simulink model "final_heart_sym2_level4_fixed"  (R2021a)
settings: Solver=VariableStepAuto  StartTime=0.0  StopTime=8  RelTol=1e-3
undefined symbols (not defined in the file or in its folder): lambda2
libraries: dspsigops x1, dspquant2 x1
(part 1 of 2)
settings Model: Creator=Ruth Matienzo  LastModifiedBy=Acer

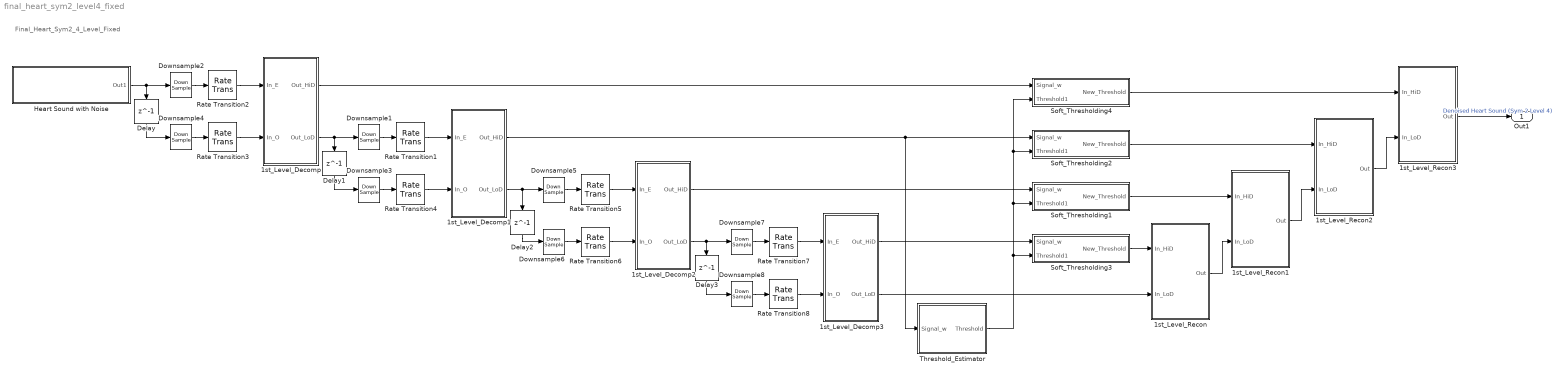
== system final_heart_sym2_level4_fixed ==
  note: Final_Heart_Sym2_4_Level_Fixed
  1st_Level_Decomp : Subsystem
  1st_Level_Decomp1 : Subsystem
  1st_Level_Decomp2 : Subsystem
  1st_Level_Decomp3 : Subsystem
  1st_Level_Recon : Subsystem
  1st_Level_Recon1 : Subsystem
  1st_Level_Recon2 : Subsystem
  1st_Level_Recon3 : Subsystem
  Delay{,1..3} (4 alike) : Delay  DelayLength=1  SampleTime=1/44100
  Downsample{1..8} (8 alike) : DownSample  N=30  RateOptions=Allow multirate processing
  Heart Sound with Noise : Subsystem
  Rate Transition{1..8} (8 alike) : RateTransition
  Soft_Thresholding1 : Subsystem
  Soft_Thresholding2 : Subsystem
  Soft_Thresholding3 : Subsystem
  Soft_Thresholding4 : Subsystem
  Threshold_Estimator : Subsystem
  Out1 : Outport  OutDataTypeStr=double  SampleTime=1/44100
  wires:
  1st_Level_Decomp1/1(Out_HiD) -> Soft_Thresholding2/1(Signal_w), Threshold_Estimator/1(Signal_w)
  1st_Level_Decomp/1(Out_HiD) -> Soft_Thresholding4/1(Signal_w)
  Delay1/1 -> Downsample3/1
  1st_Level_Decomp/2(Out_LoD) -> Downsample1/1, Delay1/1
  1st_Level_Decomp1/2(Out_LoD) -> Downsample5/1, Delay2/1
  Delay2/1 -> Downsample6/1
  Soft_Thresholding1/1(New_Threshold) -> 1st_Level_Recon1/1(In_HiD)
  1st_Level_Recon1/1(Out) -> 1st_Level_Recon2/2(In_LoD)
  1st_Level_Recon2/1(Out) -> 1st_Level_Recon3/2(In_LoD)
  Soft_Thresholding4/1(New_Threshold) -> 1st_Level_Recon3/1(In_HiD)
  Soft_Thresholding2/1(New_Threshold) -> 1st_Level_Recon2/1(In_HiD)
  Delay3/1 -> Downsample8/1
  1st_Level_Decomp2/1(Out_HiD) -> Soft_Thresholding1/1(Signal_w)
  1st_Level_Decomp3/1(Out_HiD) -> Soft_Thresholding3/1(Signal_w)
  Soft_Thresholding3/1(New_Threshold) -> 1st_Level_Recon/1(In_HiD)
  1st_Level_Decomp3/2(Out_LoD) -> 1st_Level_Recon/2(In_LoD)
  1st_Level_Recon/1(Out) -> 1st_Level_Recon1/2(In_LoD)
  Threshold_Estimator/1(Threshold) -> Soft_Thresholding3/2(Threshold1), Soft_Thresholding1/2(Threshold1), Soft_Thresholding4/2(Threshold1), Soft_Thresholding2/2(Threshold1)
  1st_Level_Decomp2/2(Out_LoD) -> Downsample7/1, Delay3/1
  1st_Level_Recon3/1(Out) -> Out1/1  "Denoised Heart Sound (Sym 2 Level 4)"
  Rate Transition2/1 -> 1st_Level_Decomp/1(In_E)
  Downsample2/1 -> Rate Transition2/1
  Rate Transition3/1 -> 1st_Level_Decomp/2(In_O)
  Delay/1 -> Downsample4/1
  Downsample4/1 -> Rate Transition3/1
  Heart Sound with Noise/1(Out1) -> Delay/1, Downsample2/1
  Rate Transition1/1 -> 1st_Level_Decomp1/1(In_E)
  Downsample1/1 -> Rate Transition1/1
  Rate Transition4/1 -> 1st_Level_Decomp1/2(In_O)
  Downsample3/1 -> Rate Transition4/1
  Rate Transition5/1 -> 1st_Level_Decomp2/1(In_E)
  Rate Transition6/1 -> 1st_Level_Decomp2/2(In_O)
  Downsample5/1 -> Rate Transition5/1
  Downsample6/1 -> Rate Transition6/1
  Rate Transition7/1 -> 1st_Level_Decomp3/1(In_E)
  Rate Transition8/1 -> 1st_Level_Decomp3/2(In_O)
  Downsample7/1 -> Rate Transition7/1
  Downsample8/1 -> Rate Transition8/1

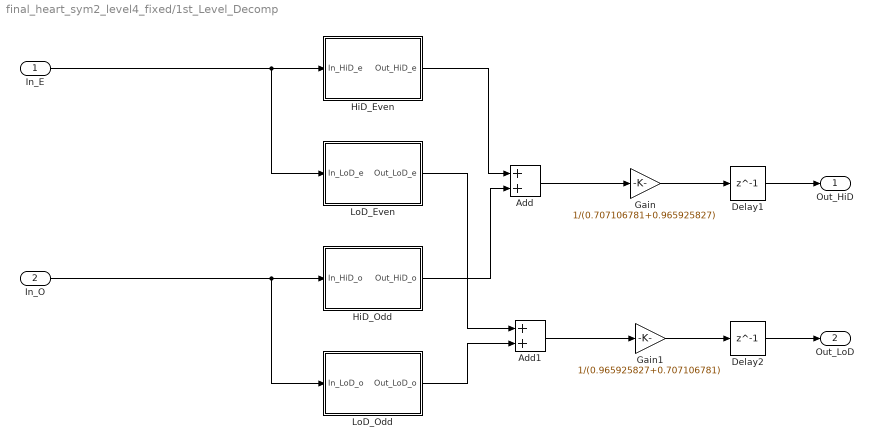
== system final_heart_sym2_level4_fixed/1st_Level_Decomp ==
  In_E : Inport  OutDataTypeStr=double  SampleTime=1/44100
  In_O : Inport  Port=2  OutDataTypeStr=double  SampleTime=1/44100
  Add : Sum  AccumDataTypeStr=double  OutDataTypeStr=double
  Add1 : Sum  AccumDataTypeStr=double  OutDataTypeStr=double
  Delay1 : Delay  DelayLength=1  SampleTime=1/44100
  Delay2 : Delay  DelayLength=1  SampleTime=1/44100
  Gain : Gain  Gain=1/(0.707106781+0.965925827)  ParamDataTypeStr=double  OutDataTypeStr=double
  Gain1 : Gain  Gain=1/(0.965925827+0.707106781)  ParamDataTypeStr=double  OutDataTypeStr=double
  HiD_Even : Subsystem
  HiD_Odd : Subsystem
  LoD_Even : Subsystem
  LoD_Odd : Subsystem
  Out_HiD : Outport  OutDataTypeStr=double  SampleTime=1/44100
  Out_LoD : Outport  Port=2  OutDataTypeStr=double  SampleTime=1/44100
  wires:
  HiD_Even/1(Out_HiD_e) -> Add/1
  HiD_Odd/1(Out_HiD_o) -> Add/2
  LoD_Even/1(Out_LoD_e) -> Add1/1
  Delay1/1 -> Out_HiD/1
  Delay2/1 -> Out_LoD/1
  In_E/1 -> HiD_Even/1(In_HiD_e), LoD_Even/1(In_LoD_e)
  In_O/1 -> HiD_Odd/1(In_HiD_o), LoD_Odd/1(In_LoD_o)
  LoD_Odd/1(Out_LoD_o) -> Add1/2
  Gain/1 -> Delay1/1
  Add/1 -> Gain/1
  Gain1/1 -> Delay2/1
  Add1/1 -> Gain1/1

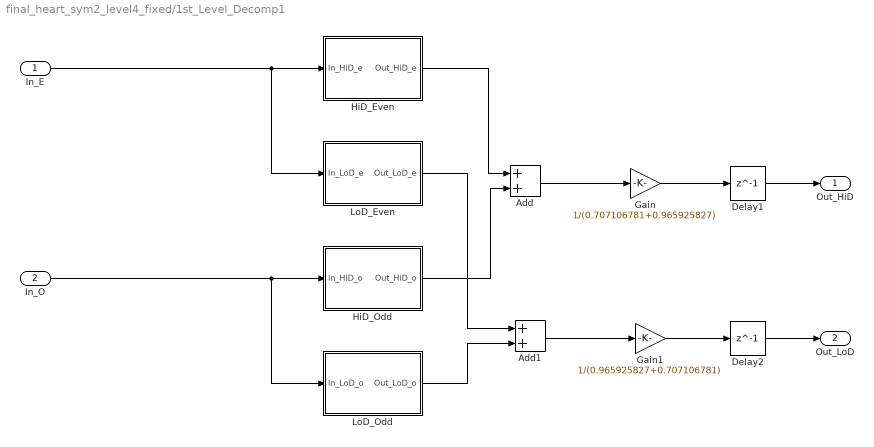
== system final_heart_sym2_level4_fixed/1st_Level_Decomp1 ==
  In_E : Inport  OutDataTypeStr=double  SampleTime=1/44100
  In_O : Inport  Port=2  OutDataTypeStr=double  SampleTime=1/44100
  Add : Sum  AccumDataTypeStr=double  OutDataTypeStr=double
  Add1 : Sum  AccumDataTypeStr=double  OutDataTypeStr=double
  Delay1 : Delay  DelayLength=1  SampleTime=1/44100
  Delay2 : Delay  DelayLength=1  SampleTime=1/44100
  Gain : Gain  Gain=1/(0.707106781+0.965925827)  ParamDataTypeStr=double  OutDataTypeStr=double
  Gain1 : Gain  Gain=1/(0.965925827+0.707106781)  ParamDataTypeStr=double  OutDataTypeStr=double
  HiD_Even : Subsystem
  HiD_Odd : Subsystem
  LoD_Even : Subsystem
  LoD_Odd : Subsystem
  Out_HiD : Outport  OutDataTypeStr=double  SampleTime=1/44100
  Out_LoD : Outport  Port=2  OutDataTypeStr=double  SampleTime=1/44100
  wires:
  HiD_Even/1(Out_HiD_e) -> Add/1
  HiD_Odd/1(Out_HiD_o) -> Add/2
  LoD_Even/1(Out_LoD_e) -> Add1/1
  Delay1/1 -> Out_HiD/1
  Delay2/1 -> Out_LoD/1
  In_E/1 -> HiD_Even/1(In_HiD_e), LoD_Even/1(In_LoD_e)
  In_O/1 -> HiD_Odd/1(In_HiD_o), LoD_Odd/1(In_LoD_o)
  LoD_Odd/1(Out_LoD_o) -> Add1/2
  Gain/1 -> Delay1/1
  Add/1 -> Gain/1
  Gain1/1 -> Delay2/1
  Add1/1 -> Gain1/1

== system final_heart_sym2_level4_fixed/1st_Level_Decomp2 ==
  In_E : Inport  OutDataTypeStr=double  SampleTime=1/44100
  In_O : Inport  Port=2  OutDataTypeStr=double  SampleTime=1/44100
  Add : Sum  AccumDataTypeStr=double  OutDataTypeStr=double
  Add1 : Sum  AccumDataTypeStr=double  OutDataTypeStr=double
  Delay1 : Delay  DelayLength=1  SampleTime=1/44100
  Delay2 : Delay  DelayLength=1  SampleTime=1/44100
  Gain : Gain  Gain=1/(0.707106781+0.965925827)  ParamDataTypeStr=double  OutDataTypeStr=double
  Gain1 : Gain  Gain=1/(0.965925827+0.707106781)  ParamDataTypeStr=double  OutDataTypeStr=double
  HiD_Even : Subsystem
  HiD_Odd : Subsystem
  LoD_Even : Subsystem
  LoD_Odd : Subsystem
  Out_HiD : Outport  OutDataTypeStr=double  SampleTime=1/44100
  Out_LoD : Outport  Port=2  OutDataTypeStr=double  SampleTime=1/44100
  wires:
  HiD_Even/1(Out_HiD_e) -> Add/1
  HiD_Odd/1(Out_HiD_o) -> Add/2
  LoD_Even/1(Out_LoD_e) -> Add1/1
  Delay1/1 -> Out_HiD/1
  Delay2/1 -> Out_LoD/1
  In_E/1 -> HiD_Even/1(In_HiD_e), LoD_Even/1(In_LoD_e)
  In_O/1 -> HiD_Odd/1(In_HiD_o), LoD_Odd/1(In_LoD_o)
  LoD_Odd/1(Out_LoD_o) -> Add1/2
  Gain/1 -> Delay1/1
  Add/1 -> Gain/1
  Gain1/1 -> Delay2/1
  Add1/1 -> Gain1/1

== system final_heart_sym2_level4_fixed/1st_Level_Decomp3 ==
  In_E : Inport  OutDataTypeStr=double  SampleTime=1/44100
  In_O : Inport  Port=2  OutDataTypeStr=double  SampleTime=1/44100
  Add : Sum  AccumDataTypeStr=double  OutDataTypeStr=double
  Add1 : Sum  AccumDataTypeStr=double  OutDataTypeStr=double
  Delay1 : Delay  DelayLength=1  SampleTime=1/44100
  Delay2 : Delay  DelayLength=1  SampleTime=1/44100
  Gain : Gain  Gain=1/(0.707106781+0.965925827)  ParamDataTypeStr=double  OutDataTypeStr=double
  Gain1 : Gain  Gain=1/(0.965925827+0.707106781)  ParamDataTypeStr=double  OutDataTypeStr=double
  HiD_Even : Subsystem
  HiD_Odd : Subsystem
  LoD_Even : Subsystem
  LoD_Odd : Subsystem
  Out_HiD : Outport  OutDataTypeStr=double  SampleTime=1/44100
  Out_LoD : Outport  Port=2  OutDataTypeStr=double  SampleTime=1/44100
  wires:
  HiD_Even/1(Out_HiD_e) -> Add/1
  HiD_Odd/1(Out_HiD_o) -> Add/2
  LoD_Even/1(Out_LoD_e) -> Add1/1
  Delay1/1 -> Out_HiD/1
  Delay2/1 -> Out_LoD/1
  In_E/1 -> HiD_Even/1(In_HiD_e), LoD_Even/1(In_LoD_e)
  In_O/1 -> HiD_Odd/1(In_HiD_o), LoD_Odd/1(In_LoD_o)
  LoD_Odd/1(Out_LoD_o) -> Add1/2
  Gain/1 -> Delay1/1
  Add/1 -> Gain/1
  Gain1/1 -> Delay2/1
  Add1/1 -> Gain1/1

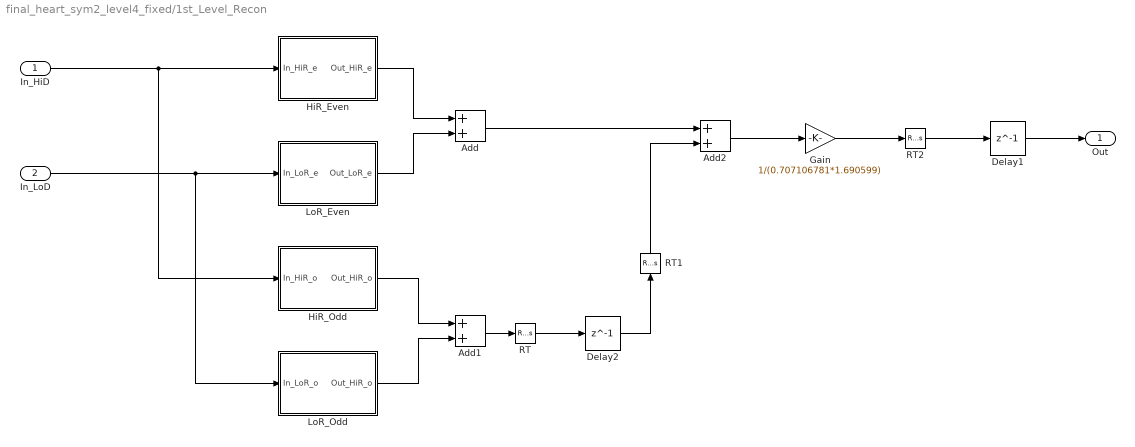
== system final_heart_sym2_level4_fixed/1st_Level_Recon ==
  In_HiD : Inport  OutDataTypeStr=double  SampleTime=1/44100
  In_LoD : Inport  Port=2  OutDataTypeStr=double  SampleTime=1/44100
  Add : Sum  AccumDataTypeStr=double  OutDataTypeStr=double
  Add1 : Sum  AccumDataTypeStr=double  OutDataTypeStr=double
  Add2 : Sum  AccumDataTypeStr=double  OutDataTypeStr=double
  Delay1 : Delay  DelayLength=1  SampleTime=1/44100
  Delay2 : Delay  DelayLength=1  SampleTime=1/44100
  Gain : Gain  Gain=1/(0.707106781*1.690599)  ParamDataTypeStr=double  OutDataTypeStr=double
  HiR_Even : Subsystem
  HiR_Odd : Subsystem
  LoR_Even : Subsystem
  LoR_Odd : Subsystem
  RT : RateTransition
  RT1 : RateTransition
  RT2 : RateTransition
  Out : Outport  OutDataTypeStr=double  SampleTime=1/44100
  wires:
  LoR_Odd/1(Out_HiR_o) -> Add1/2
  In_HiD/1 -> HiR_Even/1(In_HiR_e), HiR_Odd/1(In_HiR_o)
  In_LoD/1 -> LoR_Odd/1(In_LoR_o), LoR_Even/1(In_LoR_e)
  HiR_Even/1(Out_HiR_e) -> Add/1
  LoR_Even/1(Out_LoR_e) -> Add/2
  HiR_Odd/1(Out_HiR_o) -> Add1/1
  Delay1/1 -> Out/1
  Delay2/1 -> RT1/1
  RT2/1 -> Delay1/1
  RT1/1 -> Add2/2
  RT/1 -> Delay2/1
  Gain/1 -> RT2/1
  Add2/1 -> Gain/1
  Add/1 -> Add2/1
  Add1/1 -> RT/1

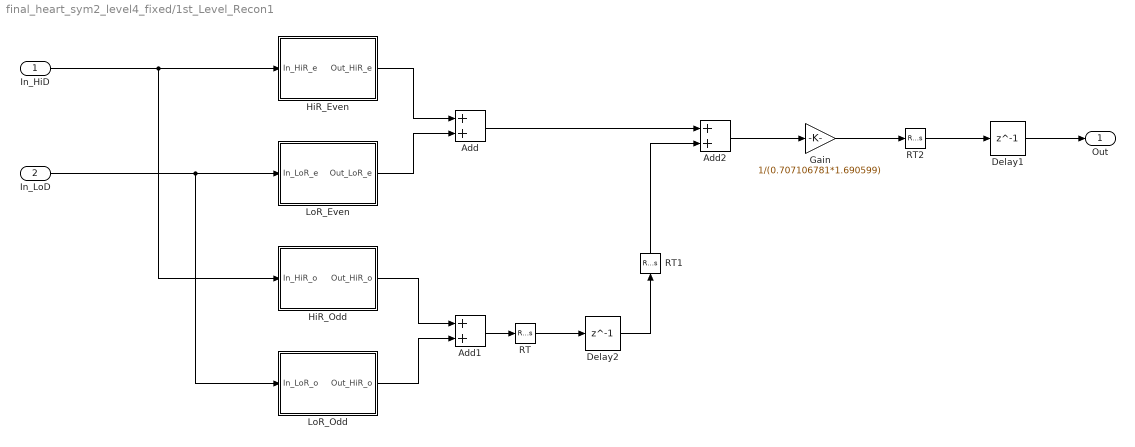
== system final_heart_sym2_level4_fixed/1st_Level_Recon1 ==
  In_HiD : Inport  OutDataTypeStr=double  SampleTime=1/44100
  In_LoD : Inport  Port=2  OutDataTypeStr=double  SampleTime=1/44100
  Add : Sum  AccumDataTypeStr=double  OutDataTypeStr=double
  Add1 : Sum  AccumDataTypeStr=double  OutDataTypeStr=double
  Add2 : Sum  AccumDataTypeStr=double  OutDataTypeStr=double
  Delay1 : Delay  DelayLength=1  SampleTime=1/44100
  Delay2 : Delay  DelayLength=1  SampleTime=1/44100
  Gain : Gain  Gain=1/(0.707106781*1.690599)  ParamDataTypeStr=double  OutDataTypeStr=double
  HiR_Even : Subsystem
  HiR_Odd : Subsystem
  LoR_Even : Subsystem
  LoR_Odd : Subsystem
  RT : RateTransition
  RT1 : RateTransition
  RT2 : RateTransition
  Out : Outport  OutDataTypeStr=double  SampleTime=1/44100
  wires:
  LoR_Odd/1(Out_HiR_o) -> Add1/2
  In_HiD/1 -> HiR_Even/1(In_HiR_e), HiR_Odd/1(In_HiR_o)
  In_LoD/1 -> LoR_Odd/1(In_LoR_o), LoR_Even/1(In_LoR_e)
  HiR_Even/1(Out_HiR_e) -> Add/1
  LoR_Even/1(Out_LoR_e) -> Add/2
  HiR_Odd/1(Out_HiR_o) -> Add1/1
  Delay1/1 -> Out/1
  Delay2/1 -> RT1/1
  RT2/1 -> Delay1/1
  RT1/1 -> Add2/2
  RT/1 -> Delay2/1
  Gain/1 -> RT2/1
  Add2/1 -> Gain/1
  Add/1 -> Add2/1
  Add1/1 -> RT/1

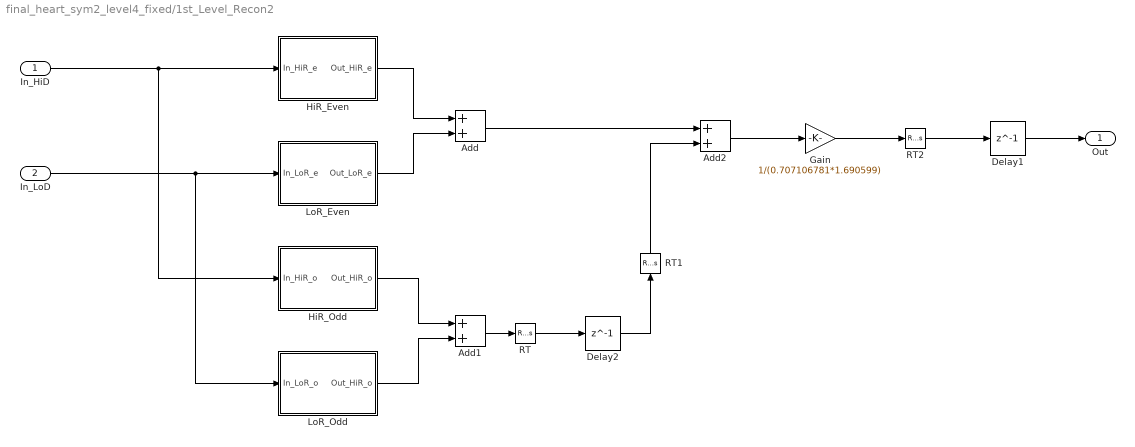
== system final_heart_sym2_level4_fixed/1st_Level_Recon2 ==
  In_HiD : Inport  OutDataTypeStr=double  SampleTime=1/44100
  In_LoD : Inport  Port=2  OutDataTypeStr=double  SampleTime=1/44100
  Add : Sum  AccumDataTypeStr=double  OutDataTypeStr=double
  Add1 : Sum  AccumDataTypeStr=double  OutDataTypeStr=double
  Add2 : Sum  AccumDataTypeStr=double  OutDataTypeStr=double
  Delay1 : Delay  DelayLength=1  SampleTime=1/44100
  Delay2 : Delay  DelayLength=1  SampleTime=1/44100
  Gain : Gain  Gain=1/(0.707106781*1.690599)  ParamDataTypeStr=double  OutDataTypeStr=double
  HiR_Even : Subsystem
  HiR_Odd : Subsystem
  LoR_Even : Subsystem
  LoR_Odd : Subsystem
  RT : RateTransition
  RT1 : RateTransition
  RT2 : RateTransition
  Out : Outport  OutDataTypeStr=double  SampleTime=1/44100
  wires:
  LoR_Odd/1(Out_HiR_o) -> Add1/2
  In_HiD/1 -> HiR_Even/1(In_HiR_e), HiR_Odd/1(In_HiR_o)
  In_LoD/1 -> LoR_Odd/1(In_LoR_o), LoR_Even/1(In_LoR_e)
  HiR_Even/1(Out_HiR_e) -> Add/1
  LoR_Even/1(Out_LoR_e) -> Add/2
  HiR_Odd/1(Out_HiR_o) -> Add1/1
  Delay1/1 -> Out/1
  Delay2/1 -> RT1/1
  RT2/1 -> Delay1/1
  RT1/1 -> Add2/2
  RT/1 -> Delay2/1
  Gain/1 -> RT2/1
  Add2/1 -> Gain/1
  Add/1 -> Add2/1
  Add1/1 -> RT/1

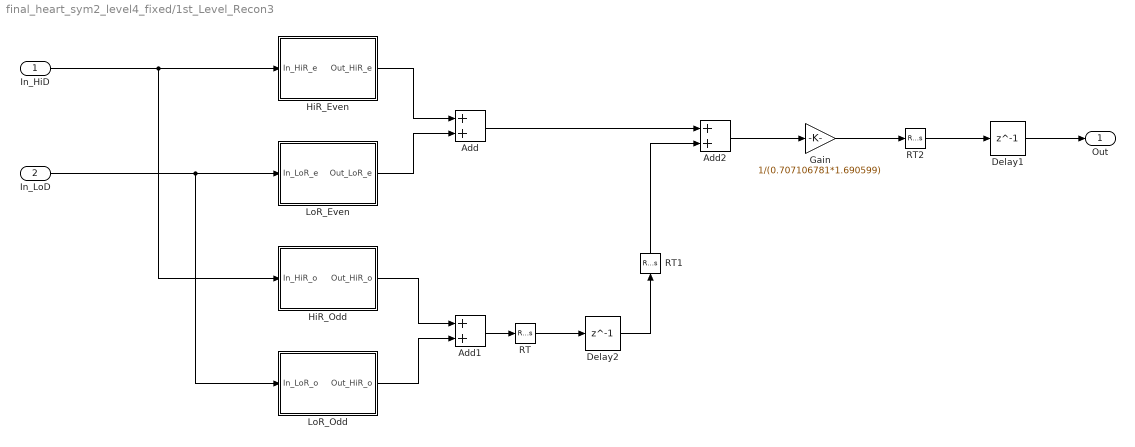
== system final_heart_sym2_level4_fixed/1st_Level_Recon3 ==
  In_HiD : Inport  OutDataTypeStr=double  SampleTime=1/44100
  In_LoD : Inport  Port=2  OutDataTypeStr=double  SampleTime=1/44100
  Add : Sum  AccumDataTypeStr=double  OutDataTypeStr=double
  Add1 : Sum  AccumDataTypeStr=double  OutDataTypeStr=double
  Add2 : Sum  AccumDataTypeStr=double  OutDataTypeStr=double
  Delay1 : Delay  DelayLength=1  SampleTime=1/44100
  Delay2 : Delay  DelayLength=1  SampleTime=1/44100
  Gain : Gain  Gain=1/(0.707106781*1.690599)  ParamDataTypeStr=double  OutDataTypeStr=double
  HiR_Even : Subsystem
  HiR_Odd : Subsystem
  LoR_Even : Subsystem
  LoR_Odd : Subsystem
  RT : RateTransition
  RT1 : RateTransition
  RT2 : RateTransition
  Out : Outport  OutDataTypeStr=double  SampleTime=1/44100
  wires:
  LoR_Odd/1(Out_HiR_o) -> Add1/2
  In_HiD/1 -> HiR_Even/1(In_HiR_e), HiR_Odd/1(In_HiR_o)
  In_LoD/1 -> LoR_Odd/1(In_LoR_o), LoR_Even/1(In_LoR_e)
  HiR_Even/1(Out_HiR_e) -> Add/1
  LoR_Even/1(Out_LoR_e) -> Add/2
  HiR_Odd/1(Out_HiR_o) -> Add1/1
  Delay1/1 -> Out/1
  Delay2/1 -> RT1/1
  RT2/1 -> Delay1/1
  RT1/1 -> Add2/2
  RT/1 -> Delay2/1
  Gain/1 -> RT2/1
  Add2/1 -> Gain/1
  Add/1 -> Add2/1
  Add1/1 -> RT/1

== system final_heart_sym2_level4_fixed/Heart Sound with Noise ==
  Constant : Constant  Value=80000  OutDataTypeStr=double  SampleTime=1/44100
  Divide : Product  Inputs=*/  OutDataTypeStr=double
  From Workspace1 : FromWorkspace  VariableName=Audio_Heart_Noise  OutDataTypeStr=double  SampleTime=1/44100
  Gain2 : Gain  Gain=5  ParamDataTypeStr=double  OutDataTypeStr=double
  Pulse Generator : DiscretePulseGenerator  PulseType=Time based  Period=0.00022675736  PulseWidth=50
  Quantizer : Quantizer  QuantizationInterval=0.1
  Sample and Hold : dspsigops/Sample and Hold  trig=Rising edge  initCond=0  latchinput=off
  Uniform Encoder : dspquant2/Uniform Encoder  peak=2  bits=8  otype=Unsigned integer
  Out1 : Outport  OutDataTypeStr=double  SampleTime=1/44100
  wires:
  Sample and Hold/1 -> Quantizer/1
  Uniform Encoder/1 -> Divide/1
  Quantizer/1 -> Uniform Encoder/1
  Constant/1 -> Divide/2
  From Workspace1/1 -> Gain2/1
  Pulse Generator/1 -> Sample and Hold/Trigger
  Gain2/1 -> Sample and Hold/1
  Divide/1 -> Out1/1

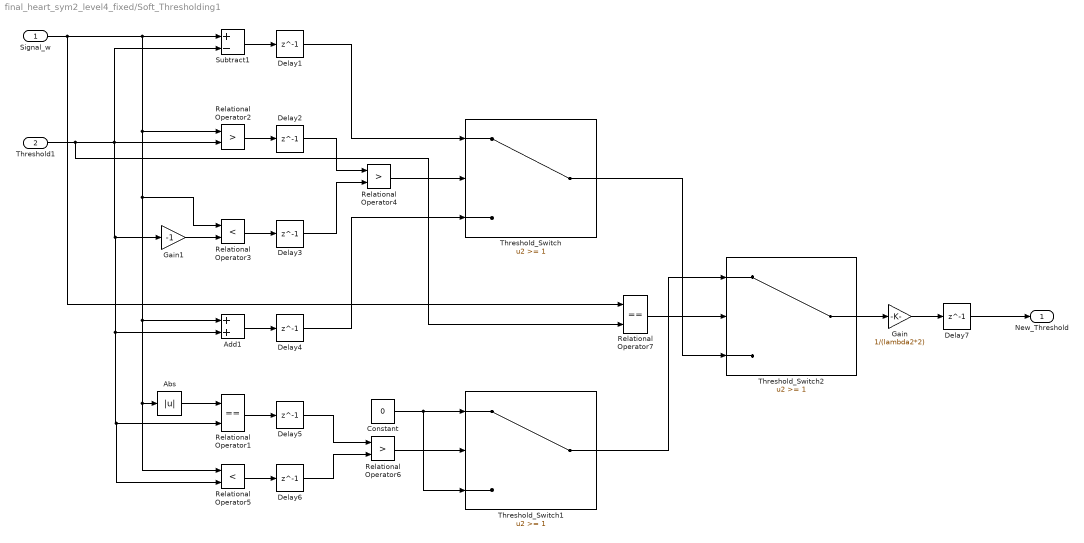
== system final_heart_sym2_level4_fixed/Soft_Thresholding1 ==
  Signal_w : Inport  OutDataTypeStr=double  SampleTime=1/44100
  Threshold1 : Inport  Port=2  OutDataTypeStr=double  SampleTime=1/44100
  Abs : Abs  OutDataTypeStr=double
  Add1 : Sum  AccumDataTypeStr=double  OutDataTypeStr=double
  Constant : Constant  Value=0  OutDataTypeStr=double  SampleTime=1/44100
  Delay{1..7} (7 alike) : Delay  DelayLength=1  SampleTime=1/44100
  Gain : Gain  Gain=1/(lambda2*2)  ParamDataTypeStr=double  OutDataTypeStr=double
  Gain1 : Gain  Gain=-1  ParamDataTypeStr=double  OutMin=-1  OutMax=-0.99  OutDataTypeStr=double
  Relational Operator1 : RelationalOperator  Operator===  OutDataTypeStr=boolean  RndMeth=Simplest
  Relational Operator2 : RelationalOperator  Operator=>  OutDataTypeStr=boolean  RndMeth=Simplest
  Relational Operator3 : RelationalOperator  Operator=<  OutDataTypeStr=boolean  RndMeth=Simplest
  Relational Operator4 : RelationalOperator  Operator=>  OutDataTypeStr=boolean  RndMeth=Simplest
  Relational Operator5 : RelationalOperator  Operator=<  OutDataTypeStr=boolean  RndMeth=Simplest
  Relational Operator6 : RelationalOperator  Operator=>  OutDataTypeStr=boolean  RndMeth=Simplest
  Relational Operator7 : RelationalOperator  Operator===  OutDataTypeStr=boolean  RndMeth=Simplest
  Subtract1 : Sum  Inputs=+-  AccumDataTypeStr=double  OutDataTypeStr=double
  Threshold_Switch : Switch  Threshold=1  OutDataTypeStr=double
  Threshold_Switch1 : Switch  Threshold=1  OutDataTypeStr=double
  Threshold_Switch2 : Switch  Threshold=1  OutDataTypeStr=double
  New_Threshold : Outport  OutDataTypeStr=double  SampleTime=1/44100
  wires:
  Threshold_Switch/1 -> Threshold_Switch2/3
  Relational Operator6/1 -> Threshold_Switch1/2
  Gain1/1 -> Relational Operator3/2
  Delay4/1 -> Threshold_Switch/3
  Add1/1 -> Delay4/1
  Delay2/1 -> Relational Operator4/1
  Delay3/1 -> Relational Operator4/2
  Delay1/1 -> Threshold_Switch/1
  Relational Operator2/1 -> Delay2/1
  Relational Operator3/1 -> Delay3/1
  Relational Operator5/1 -> Delay6/1
  Delay6/1 -> Relational Operator6/2
  Delay5/1 -> Relational Operator6/1
  Threshold1/1 -> Relational Operator2/2, Subtract1/2, Relational Operator5/2, Relational Operator1/2, Add1/2, Gain1/1, Relational Operator7/2
  Abs/1 -> Relational Operator1/1
  Relational Operator4/1 -> Threshold_Switch/2
  Subtract1/1 -> Delay1/1
  Constant/1 -> Threshold_Switch1/3, Threshold_Switch1/1
  Signal_w/1 -> Subtract1/1, Relational Operator2/1, Relational Operator5/1, Abs/1, Add1/1, Relational Operator3/1, Relational Operator7/1
  Relational Operator7/1 -> Threshold_Switch2/2
  Relational Operator1/1 -> Delay5/1
  Threshold_Switch1/1 -> Threshold_Switch2/1
  Delay7/1 -> New_Threshold/1
  Threshold_Switch2/1 -> Gain/1
  Gain/1 -> Delay7/1

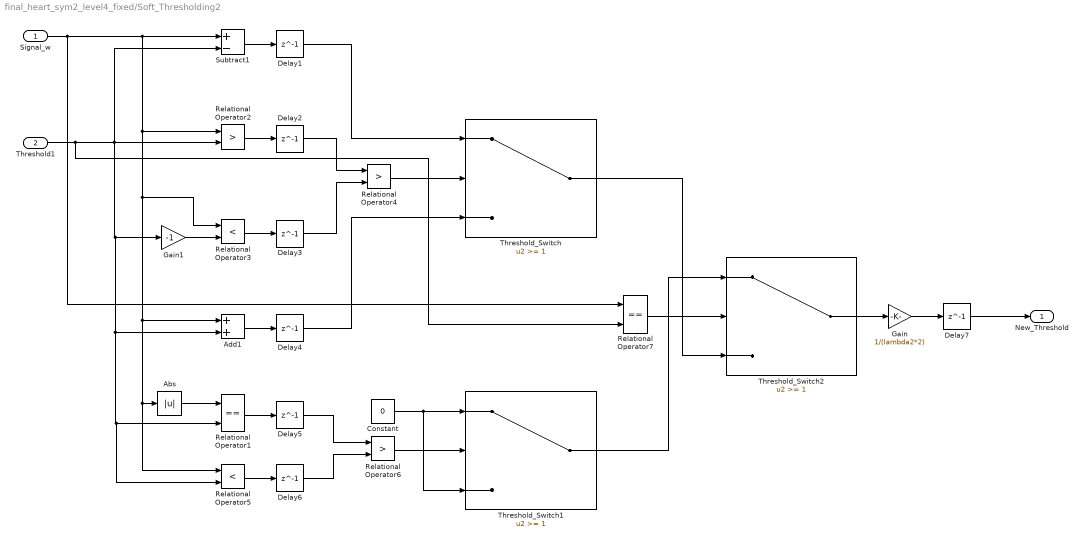
== system final_heart_sym2_level4_fixed/Soft_Thresholding2 ==
  Signal_w : Inport  OutDataTypeStr=double  SampleTime=1/44100
  Threshold1 : Inport  Port=2  OutDataTypeStr=double  SampleTime=1/44100
  Abs : Abs  OutDataTypeStr=double
  Add1 : Sum  AccumDataTypeStr=double  OutDataTypeStr=double
  Constant : Constant  Value=0  OutDataTypeStr=double  SampleTime=1/44100
  Delay{1..7} (7 alike) : Delay  DelayLength=1  SampleTime=1/44100
  Gain : Gain  Gain=1/(lambda2*2)  ParamDataTypeStr=double  OutDataTypeStr=double
  Gain1 : Gain  Gain=-1  ParamDataTypeStr=double  OutMin=-1  OutMax=-0.99  OutDataTypeStr=double
  Relational Operator1 : RelationalOperator  Operator===  OutDataTypeStr=boolean  RndMeth=Simplest
  Relational Operator2 : RelationalOperator  Operator=>  OutDataTypeStr=boolean  RndMeth=Simplest
  Relational Operator3 : RelationalOperator  Operator=<  OutDataTypeStr=boolean  RndMeth=Simplest
  Relational Operator4 : RelationalOperator  Operator=>  OutDataTypeStr=boolean  RndMeth=Simplest
  Relational Operator5 : RelationalOperator  Operator=<  OutDataTypeStr=boolean  RndMeth=Simplest
  Relational Operator6 : RelationalOperator  Operator=>  OutDataTypeStr=boolean  RndMeth=Simplest
  Relational Operator7 : RelationalOperator  Operator===  OutDataTypeStr=boolean  RndMeth=Simplest
  Subtract1 : Sum  Inputs=+-  AccumDataTypeStr=double  OutDataTypeStr=double
  Threshold_Switch : Switch  Threshold=1  OutDataTypeStr=double
  Threshold_Switch1 : Switch  Threshold=1  OutDataTypeStr=double
  Threshold_Switch2 : Switch  Threshold=1  OutDataTypeStr=double
  New_Threshold : Outport  OutDataTypeStr=double  SampleTime=1/44100
  wires:
  Threshold_Switch/1 -> Threshold_Switch2/3
  Relational Operator6/1 -> Threshold_Switch1/2
  Gain1/1 -> Relational Operator3/2
  Delay4/1 -> Threshold_Switch/3
  Add1/1 -> Delay4/1
  Delay2/1 -> Relational Operator4/1
  Delay3/1 -> Relational Operator4/2
  Delay1/1 -> Threshold_Switch/1
  Relational Operator2/1 -> Delay2/1
  Relational Operator3/1 -> Delay3/1
  Relational Operator5/1 -> Delay6/1
  Delay6/1 -> Relational Operator6/2
  Delay5/1 -> Relational Operator6/1
  Threshold1/1 -> Relational Operator2/2, Subtract1/2, Relational Operator5/2, Relational Operator1/2, Add1/2, Gain1/1, Relational Operator7/2
  Abs/1 -> Relational Operator1/1
  Relational Operator4/1 -> Threshold_Switch/2
  Subtract1/1 -> Delay1/1
  Constant/1 -> Threshold_Switch1/3, Threshold_Switch1/1
  Signal_w/1 -> Subtract1/1, Relational Operator2/1, Relational Operator5/1, Abs/1, Add1/1, Relational Operator3/1, Relational Operator7/1
  Relational Operator7/1 -> Threshold_Switch2/2
  Relational Operator1/1 -> Delay5/1
  Threshold_Switch1/1 -> Threshold_Switch2/1
  Delay7/1 -> New_Threshold/1
  Threshold_Switch2/1 -> Gain/1
  Gain/1 -> Delay7/1

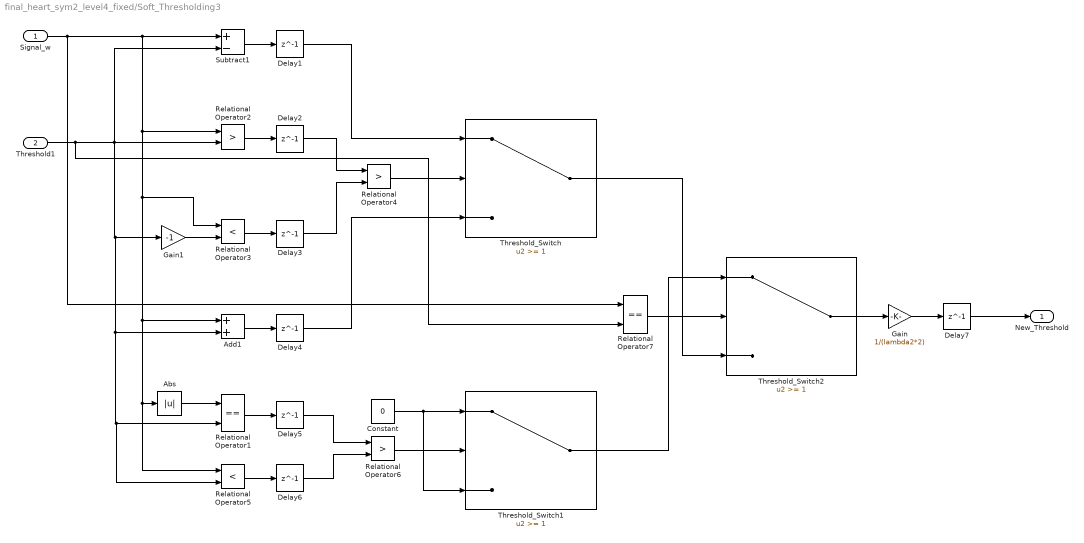
== system final_heart_sym2_level4_fixed/Soft_Thresholding3 ==
  Signal_w : Inport  OutDataTypeStr=double  SampleTime=1/44100
  Threshold1 : Inport  Port=2  OutDataTypeStr=double  SampleTime=1/44100
  Abs : Abs  OutDataTypeStr=double
  Add1 : Sum  AccumDataTypeStr=double  OutDataTypeStr=double
  Constant : Constant  Value=0  OutDataTypeStr=double  SampleTime=1/44100
  Delay{1..7} (7 alike) : Delay  DelayLength=1  SampleTime=1/44100
  Gain : Gain  Gain=1/(lambda2*2)  ParamDataTypeStr=double  OutDataTypeStr=double
  Gain1 : Gain  Gain=-1  ParamDataTypeStr=double  OutMin=-1  OutMax=-0.99  OutDataTypeStr=double
  Relational Operator1 : RelationalOperator  Operator===  OutDataTypeStr=boolean  RndMeth=Simplest
  Relational Operator2 : RelationalOperator  Operator=>  OutDataTypeStr=boolean  RndMeth=Simplest
  Relational Operator3 : RelationalOperator  Operator=<  OutDataTypeStr=boolean  RndMeth=Simplest
  Relational Operator4 : RelationalOperator  Operator=>  OutDataTypeStr=boolean  RndMeth=Simplest
  Relational Operator5 : RelationalOperator  Operator=<  OutDataTypeStr=boolean  RndMeth=Simplest
  Relational Operator6 : RelationalOperator  Operator=>  OutDataTypeStr=boolean  RndMeth=Simplest
  Relational Operator7 : RelationalOperator  Operator===  OutDataTypeStr=boolean  RndMeth=Simplest
  Subtract1 : Sum  Inputs=+-  AccumDataTypeStr=double  OutDataTypeStr=double
  Threshold_Switch : Switch  Threshold=1  OutDataTypeStr=double
  Threshold_Switch1 : Switch  Threshold=1  OutDataTypeStr=double
  Threshold_Switch2 : Switch  Threshold=1  OutDataTypeStr=double
  New_Threshold : Outport  OutDataTypeStr=double  SampleTime=1/44100
  wires:
  Threshold_Switch/1 -> Threshold_Switch2/3
  Relational Operator6/1 -> Threshold_Switch1/2
  Gain1/1 -> Relational Operator3/2
  Delay4/1 -> Threshold_Switch/3
  Add1/1 -> Delay4/1
  Delay2/1 -> Relational Operator4/1
  Delay3/1 -> Relational Operator4/2
  Delay1/1 -> Threshold_Switch/1
  Relational Operator2/1 -> Delay2/1
  Relational Operator3/1 -> Delay3/1
  Relational Operator5/1 -> Delay6/1
  Delay6/1 -> Relational Operator6/2
  Delay5/1 -> Relational Operator6/1
  Threshold1/1 -> Relational Operator2/2, Subtract1/2, Relational Operator5/2, Relational Operator1/2, Add1/2, Gain1/1, Relational Operator7/2
  Abs/1 -> Relational Operator1/1
  Relational Operator4/1 -> Threshold_Switch/2
  Subtract1/1 -> Delay1/1
  Constant/1 -> Threshold_Switch1/3, Threshold_Switch1/1
  Signal_w/1 -> Subtract1/1, Relational Operator2/1, Relational Operator5/1, Abs/1, Add1/1, Relational Operator3/1, Relational Operator7/1
  Relational Operator7/1 -> Threshold_Switch2/2
  Relational Operator1/1 -> Delay5/1
  Threshold_Switch1/1 -> Threshold_Switch2/1
  Delay7/1 -> New_Threshold/1
  Threshold_Switch2/1 -> Gain/1
  Gain/1 -> Delay7/1

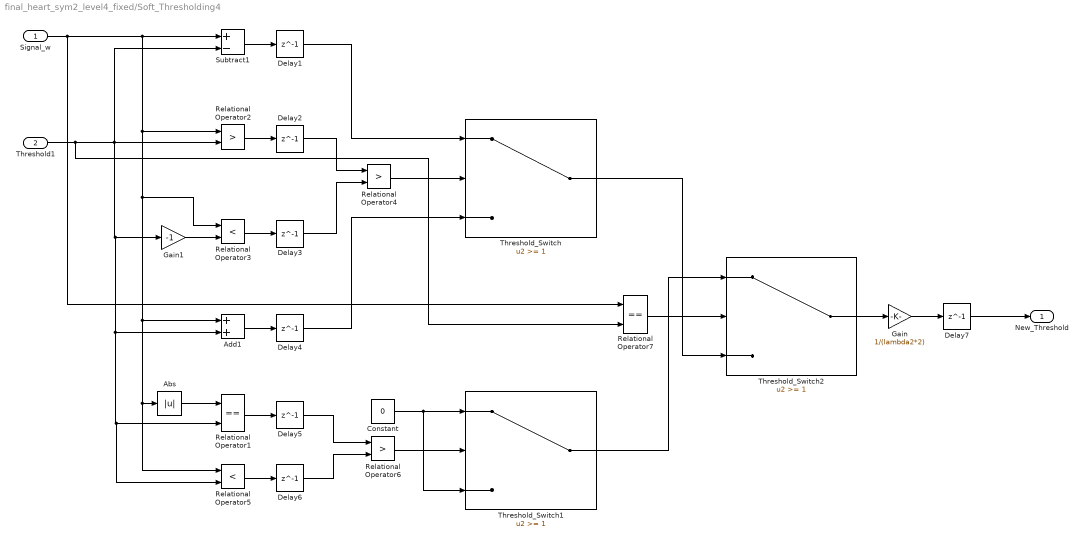
== system final_heart_sym2_level4_fixed/Soft_Thresholding4 ==
  Signal_w : Inport  OutDataTypeStr=double  SampleTime=1/44100
  Threshold1 : Inport  Port=2  OutDataTypeStr=double  SampleTime=1/44100
  Abs : Abs  OutDataTypeStr=double
  Add1 : Sum  AccumDataTypeStr=double  OutDataTypeStr=double
  Constant : Constant  Value=0  OutDataTypeStr=double  SampleTime=1/44100
  Delay{1..7} (7 alike) : Delay  DelayLength=1  SampleTime=1/44100
  Gain : Gain  Gain=1/(lambda2*2)  ParamDataTypeStr=double  OutDataTypeStr=double
  Gain1 : Gain  Gain=-1  ParamDataTypeStr=double  OutMin=-1  OutMax=-0.99  OutDataTypeStr=double
  Relational Operator1 : RelationalOperator  Operator===  OutDataTypeStr=boolean  RndMeth=Simplest
  Relational Operator2 : RelationalOperator  Operator=>  OutDataTypeStr=boolean  RndMeth=Simplest
  Relational Operator3 : RelationalOperator  Operator=<  OutDataTypeStr=boolean  RndMeth=Simplest
  Relational Operator4 : RelationalOperator  Operator=>  OutDataTypeStr=boolean  RndMeth=Simplest
  Relational Operator5 : RelationalOperator  Operator=<  OutDataTypeStr=boolean  RndMeth=Simplest
  Relational Operator6 : RelationalOperator  Operator=>  OutDataTypeStr=boolean  RndMeth=Simplest
  Relational Operator7 : RelationalOperator  Operator===  OutDataTypeStr=boolean  RndMeth=Simplest
  Subtract1 : Sum  Inputs=+-  AccumDataTypeStr=double  OutDataTypeStr=double
  Threshold_Switch : Switch  Threshold=1  OutDataTypeStr=double
  Threshold_Switch1 : Switch  Threshold=1  OutDataTypeStr=double
  Threshold_Switch2 : Switch  Threshold=1  OutDataTypeStr=double
  New_Threshold : Outport  OutDataTypeStr=double  SampleTime=1/44100
  wires:
  Threshold_Switch/1 -> Threshold_Switch2/3
  Relational Operator6/1 -> Threshold_Switch1/2
  Gain1/1 -> Relational Operator3/2
  Delay4/1 -> Threshold_Switch/3
  Add1/1 -> Delay4/1
  Delay2/1 -> Relational Operator4/1
  Delay3/1 -> Relational Operator4/2
  Delay1/1 -> Threshold_Switch/1
  Relational Operator2/1 -> Delay2/1
  Relational Operator3/1 -> Delay3/1
  Relational Operator5/1 -> Delay6/1
  Delay6/1 -> Relational Operator6/2
  Delay5/1 -> Relational Operator6/1
  Threshold1/1 -> Relational Operator2/2, Subtract1/2, Relational Operator5/2, Relational Operator1/2, Add1/2, Gain1/1, Relational Operator7/2
  Abs/1 -> Relational Operator1/1
  Relational Operator4/1 -> Threshold_Switch/2
  Subtract1/1 -> Delay1/1
  Constant/1 -> Threshold_Switch1/3, Threshold_Switch1/1
  Signal_w/1 -> Subtract1/1, Relational Operator2/1, Relational Operator5/1, Abs/1, Add1/1, Relational Operator3/1, Relational Operator7/1
  Relational Operator7/1 -> Threshold_Switch2/2
  Relational Operator1/1 -> Delay5/1
  Threshold_Switch1/1 -> Threshold_Switch2/1
  Delay7/1 -> New_Threshold/1
  Threshold_Switch2/1 -> Gain/1
  Gain/1 -> Delay7/1

== system final_heart_sym2_level4_fixed/Threshold_Estimator ==
  Signal_w : Inport  OutDataTypeStr=double  SampleTime=1/44100
  Absolute_Value1 : Subsystem
  Length : Constant  Value=lambda2  OutDataTypeStr=double  SampleTime=1/44100
  Median2 : Subsystem
  Multiply : Product  OutDataTypeStr=double
  Threshold : Outport  OutDataTypeStr=double  SampleTime=1/44100  VectorParamsAs1DForOutWhenUnconnected=off
  wires:
  Length/1 -> Multiply/2
  Median2/1(Median) -> Multiply/1
  Absolute_Value1/1(Out_Abs) -> Median2/1(Signal_w3)
  Signal_w/1 -> Absolute_Value1/1(Signal_w4)
  Multiply/1 -> Threshold/1

== system final_heart_sym2_level4_fixed/1st_Level_Decomp/HiD_Even ==
  In_HiD_e : Inport  OutDataTypeStr=double  SampleTime=1/44100
  Add : Sum  AccumDataTypeStr=double  OutDataTypeStr=double
  Delay : Delay  DelayLength=1  SampleTime=1/44100
  Delay3 : Delay  DelayLength=1  SampleTime=1/44100
  HiD_0 : Constant  Value=-0.482962913  OutDataTypeStr=double  SampleTime=1/44100
  HiD_2 : Constant  Value=-0.224143868  OutDataTypeStr=double  SampleTime=1/44100
  Multiply : Product  OutDataTypeStr=double
  Multiply1 : Product  OutDataTypeStr=double
  Rate Transition : RateTransition
  Out_HiD_e : Outport  OutDataTypeStr=double  SampleTime=1/44100  VectorParamsAs1DForOutWhenUnconnected=off
  wires:
  Delay/1 -> Rate Transition/1
  Delay3/1 -> Add/2
  Multiply1/1 -> Delay3/1
  Multiply/1 -> Add/1
  HiD_0/1 -> Multiply/1
  HiD_2/1 -> Multiply1/1
  Add/1 -> Out_HiD_e/1
  In_HiD_e/1 -> Multiply/2, Delay/1
  Rate Transition/1 -> Multiply1/2

== system final_heart_sym2_level4_fixed/1st_Level_Decomp/HiD_Odd ==
  In_HiD_o : Inport  OutDataTypeStr=double  SampleTime=1/44100
  Add : Sum  AccumDataTypeStr=double  OutDataTypeStr=double
  Delay : Delay  DelayLength=1  SampleTime=1/44100
  Delay3 : Delay  DelayLength=1  SampleTime=1/44100
  HiD_1 : Constant  Value=0.836516304  OutDataTypeStr=double  SampleTime=1/44100
  HiD_3 : Constant  Value=-0.129409523  OutDataTypeStr=double  SampleTime=1/44100
  Multiply : Product  OutDataTypeStr=double
  Multiply1 : Product  OutDataTypeStr=double
  Rate Transition : RateTransition
  Out_HiD_o : Outport  OutDataTypeStr=double  SampleTime=1/44100  VectorParamsAs1DForOutWhenUnconnected=off
  wires:
  Delay/1 -> Rate Transition/1
  Delay3/1 -> Add/2
  Multiply1/1 -> Delay3/1
  Multiply/1 -> Add/1
  HiD_1/1 -> Multiply/1
  HiD_3/1 -> Multiply1/1
  Add/1 -> Out_HiD_o/1
  In_HiD_o/1 -> Delay/1, Multiply/2
  Rate Transition/1 -> Multiply1/2

== system final_heart_sym2_level4_fixed/1st_Level_Decomp/LoD_Even ==
  In_LoD_e : Inport  OutDataTypeStr=double  SampleTime=1/44100
  Add : Sum  AccumDataTypeStr=double  OutDataTypeStr=double
  Delay : Delay  DelayLength=1  SampleTime=1/44100
  Delay3 : Delay  DelayLength=1  SampleTime=1/44100
  LoD_0 : Constant  Value=-0.129409523  OutDataTypeStr=double  SampleTime=1/44100
  LoD_2 : Constant  Value=0.836516304  OutDataTypeStr=double  SampleTime=1/44100
  Multiply : Product  OutDataTypeStr=double
  Multiply1 : Product  OutDataTypeStr=double
  Rate Transition : RateTransition
  Out_LoD_e : Outport  OutDataTypeStr=double  SampleTime=1/44100  VectorParamsAs1DForOutWhenUnconnected=off
  wires:
  Delay/1 -> Rate Transition/1
  Delay3/1 -> Add/2
  Multiply1/1 -> Delay3/1
  Multiply/1 -> Add/1
  LoD_0/1 -> Multiply/1
  LoD_2/1 -> Multiply1/1
  Add/1 -> Out_LoD_e/1
  In_LoD_e/1 -> Delay/1, Multiply/2
  Rate Transition/1 -> Multiply1/2

== system final_heart_sym2_level4_fixed/1st_Level_Decomp/LoD_Odd ==
  In_LoD_o : Inport  OutDataTypeStr=double  SampleTime=1/44100
  Add : Sum  AccumDataTypeStr=double  OutDataTypeStr=double
  Delay : Delay  DelayLength=1  SampleTime=1/44100
  Delay3 : Delay  DelayLength=1  SampleTime=1/44100
  LoD_1 : Constant  Value=0.224143868  OutDataTypeStr=double  SampleTime=1/44100
  LoD_3 : Constant  Value=0.482962913  OutDataTypeStr=double  SampleTime=1/44100
  Multiply : Product  OutDataTypeStr=double
  Multiply1 : Product  OutDataTypeStr=double
  Rate Transition : RateTransition
  Out_LoD_o : Outport  OutDataTypeStr=double  SampleTime=1/44100  VectorParamsAs1DForOutWhenUnconnected=off
  wires:
  Delay/1 -> Rate Transition/1
  Delay3/1 -> Add/2
  Multiply1/1 -> Delay3/1
  Multiply/1 -> Add/1
  LoD_1/1 -> Multiply/1
  LoD_3/1 -> Multiply1/1
  Add/1 -> Out_LoD_o/1
  In_LoD_o/1 -> Delay/1, Multiply/2
  Rate Transition/1 -> Multiply1/2

== system final_heart_sym2_level4_fixed/1st_Level_Decomp1/HiD_Even ==
  In_HiD_e : Inport  OutDataTypeStr=double  SampleTime=1/44100
  Add : Sum  AccumDataTypeStr=double  OutDataTypeStr=double
  Delay : Delay  DelayLength=1  SampleTime=1/44100
  Delay3 : Delay  DelayLength=1  SampleTime=1/44100
  HiD_0 : Constant  Value=-0.482962913  OutDataTypeStr=double  SampleTime=1/44100
  HiD_2 : Constant  Value=-0.224143868  OutDataTypeStr=double  SampleTime=1/44100
  Multiply : Product  OutDataTypeStr=double
  Multiply1 : Product  OutDataTypeStr=double
  Rate Transition : RateTransition
  Out_HiD_e : Outport  OutDataTypeStr=double  SampleTime=1/44100  VectorParamsAs1DForOutWhenUnconnected=off
  wires:
  Delay/1 -> Rate Transition/1
  Delay3/1 -> Add/2
  Multiply1/1 -> Delay3/1
  Multiply/1 -> Add/1
  HiD_0/1 -> Multiply/1
  HiD_2/1 -> Multiply1/1
  Add/1 -> Out_HiD_e/1
  In_HiD_e/1 -> Multiply/2, Delay/1
  Rate Transition/1 -> Multiply1/2

== system final_heart_sym2_level4_fixed/1st_Level_Decomp1/HiD_Odd ==
  In_HiD_o : Inport  OutDataTypeStr=double  SampleTime=1/44100
  Add : Sum  AccumDataTypeStr=double  OutDataTypeStr=double
  Delay : Delay  DelayLength=1  SampleTime=1/44100
  Delay3 : Delay  DelayLength=1  SampleTime=1/44100
  HiD_1 : Constant  Value=0.836516304  OutDataTypeStr=double  SampleTime=1/44100
  HiD_3 : Constant  Value=-0.129409523  OutDataTypeStr=double  SampleTime=1/44100
  Multiply : Product  OutDataTypeStr=double
  Multiply1 : Product  OutDataTypeStr=double
  Rate Transition : RateTransition
  Out_HiD_o : Outport  OutDataTypeStr=double  SampleTime=1/44100  VectorParamsAs1DForOutWhenUnconnected=off
  wires:
  Delay/1 -> Rate Transition/1
  Delay3/1 -> Add/2
  Multiply1/1 -> Delay3/1
  Multiply/1 -> Add/1
  HiD_1/1 -> Multiply/1
  HiD_3/1 -> Multiply1/1
  Add/1 -> Out_HiD_o/1
  In_HiD_o/1 -> Delay/1, Multiply/2
  Rate Transition/1 -> Multiply1/2

== system final_heart_sym2_level4_fixed/1st_Level_Decomp1/LoD_Even ==
  In_LoD_e : Inport  OutDataTypeStr=double  SampleTime=1/44100
  Add : Sum  AccumDataTypeStr=double  OutDataTypeStr=double
  Delay : Delay  DelayLength=1  SampleTime=1/44100
  Delay3 : Delay  DelayLength=1  SampleTime=1/44100
  LoD_0 : Constant  Value=-0.129409523  OutDataTypeStr=double  SampleTime=1/44100
  LoD_2 : Constant  Value=0.836516304  OutDataTypeStr=double  SampleTime=1/44100
  Multiply : Product  OutDataTypeStr=double
  Multiply1 : Product  OutDataTypeStr=double
  Rate Transition : RateTransition
  Out_LoD_e : Outport  OutDataTypeStr=double  SampleTime=1/44100  VectorParamsAs1DForOutWhenUnconnected=off
  wires:
  Delay/1 -> Rate Transition/1
  Delay3/1 -> Add/2
  Multiply1/1 -> Delay3/1
  Multiply/1 -> Add/1
  LoD_0/1 -> Multiply/1
  LoD_2/1 -> Multiply1/1
  Add/1 -> Out_LoD_e/1
  In_LoD_e/1 -> Delay/1, Multiply/2
  Rate Transition/1 -> Multiply1/2

== system final_heart_sym2_level4_fixed/1st_Level_Decomp1/LoD_Odd ==
  In_LoD_o : Inport  OutDataTypeStr=double  SampleTime=1/44100
  Add : Sum  AccumDataTypeStr=double  OutDataTypeStr=double
  Delay : Delay  DelayLength=1  SampleTime=1/44100
  Delay3 : Delay  DelayLength=1  SampleTime=1/44100
  LoD_1 : Constant  Value=0.224143868  OutDataTypeStr=double  SampleTime=1/44100
  LoD_3 : Constant  Value=0.482962913  OutDataTypeStr=double  SampleTime=1/44100
  Multiply : Product  OutDataTypeStr=double
  Multiply1 : Product  OutDataTypeStr=double
  Rate Transition : RateTransition
  Out_LoD_o : Outport  OutDataTypeStr=double  SampleTime=1/44100  VectorParamsAs1DForOutWhenUnconnected=off
  wires:
  Delay/1 -> Rate Transition/1
  Delay3/1 -> Add/2
  Multiply1/1 -> Delay3/1
  Multiply/1 -> Add/1
  LoD_1/1 -> Multiply/1
  LoD_3/1 -> Multiply1/1
  Add/1 -> Out_LoD_o/1
  In_LoD_o/1 -> Delay/1, Multiply/2
  Rate Transition/1 -> Multiply1/2

== system final_heart_sym2_level4_fixed/1st_Level_Decomp2/HiD_Even ==
  In_HiD_e : Inport  OutDataTypeStr=double  SampleTime=1/44100
  Add : Sum  AccumDataTypeStr=double  OutDataTypeStr=double
  Delay : Delay  DelayLength=1  SampleTime=1/44100
  Delay3 : Delay  DelayLength=1  SampleTime=1/44100
  HiD_0 : Constant  Value=-0.482962913  OutDataTypeStr=double  SampleTime=1/44100
  HiD_2 : Constant  Value=-0.224143868  OutDataTypeStr=double  SampleTime=1/44100
  Multiply : Product  OutDataTypeStr=double
  Multiply1 : Product  OutDataTypeStr=double
  Rate Transition : RateTransition
  Out_HiD_e : Outport  OutDataTypeStr=double  SampleTime=1/44100  VectorParamsAs1DForOutWhenUnconnected=off
  wires:
  Delay/1 -> Rate Transition/1
  Delay3/1 -> Add/2
  Multiply1/1 -> Delay3/1
  Multiply/1 -> Add/1
  HiD_0/1 -> Multiply/1
  HiD_2/1 -> Multiply1/1
  Add/1 -> Out_HiD_e/1
  In_HiD_e/1 -> Multiply/2, Delay/1
  Rate Transition/1 -> Multiply1/2

== system final_heart_sym2_level4_fixed/1st_Level_Decomp2/HiD_Odd ==
  In_HiD_o : Inport  OutDataTypeStr=double  SampleTime=1/44100
  Add : Sum  AccumDataTypeStr=double  OutDataTypeStr=double
  Delay : Delay  DelayLength=1  SampleTime=1/44100
  Delay3 : Delay  DelayLength=1  SampleTime=1/44100
  HiD_1 : Constant  Value=0.836516304  OutDataTypeStr=double  SampleTime=1/44100
  HiD_3 : Constant  Value=-0.129409523  OutDataTypeStr=double  SampleTime=1/44100
  Multiply : Product  OutDataTypeStr=double
  Multiply1 : Product  OutDataTypeStr=double
  Rate Transition : RateTransition
  Out_HiD_o : Outport  OutDataTypeStr=double  SampleTime=1/44100  VectorParamsAs1DForOutWhenUnconnected=off
  wires:
  Delay/1 -> Rate Transition/1
  Delay3/1 -> Add/2
  Multiply1/1 -> Delay3/1
  Multiply/1 -> Add/1
  HiD_1/1 -> Multiply/1
  HiD_3/1 -> Multiply1/1
  Add/1 -> Out_HiD_o/1
  In_HiD_o/1 -> Delay/1, Multiply/2
  Rate Transition/1 -> Multiply1/2

== system final_heart_sym2_level4_fixed/1st_Level_Decomp2/LoD_Even ==
  In_LoD_e : Inport  OutDataTypeStr=double  SampleTime=1/44100
  Add : Sum  AccumDataTypeStr=double  OutDataTypeStr=double
  Delay : Delay  DelayLength=1  SampleTime=1/44100
  Delay3 : Delay  DelayLength=1  SampleTime=1/44100
  LoD_0 : Constant  Value=-0.129409523  OutDataTypeStr=double  SampleTime=1/44100
  LoD_2 : Constant  Value=0.836516304  OutDataTypeStr=double  SampleTime=1/44100
  Multiply : Product  OutDataTypeStr=double
  Multiply1 : Product  OutDataTypeStr=double
  Rate Transition : RateTransition
  Out_LoD_e : Outport  OutDataTypeStr=double  SampleTime=1/44100  VectorParamsAs1DForOutWhenUnconnected=off
  wires:
  Delay/1 -> Rate Transition/1
  Delay3/1 -> Add/2
  Multiply1/1 -> Delay3/1
  Multiply/1 -> Add/1
  LoD_0/1 -> Multiply/1
  LoD_2/1 -> Multiply1/1
  Add/1 -> Out_LoD_e/1
  In_LoD_e/1 -> Delay/1, Multiply/2
  Rate Transition/1 -> Multiply1/2

== system final_heart_sym2_level4_fixed/1st_Level_Decomp2/LoD_Odd ==
  In_LoD_o : Inport  OutDataTypeStr=double  SampleTime=1/44100
  Add : Sum  AccumDataTypeStr=double  OutDataTypeStr=double
  Delay : Delay  DelayLength=1  SampleTime=1/44100
  Delay3 : Delay  DelayLength=1  SampleTime=1/44100
  LoD_1 : Constant  Value=0.224143868  OutDataTypeStr=double  SampleTime=1/44100
  LoD_3 : Constant  Value=0.482962913  OutDataTypeStr=double  SampleTime=1/44100
  Multiply : Product  OutDataTypeStr=double
  Multiply1 : Product  OutDataTypeStr=double
  Rate Transition : RateTransition
  Out_LoD_o : Outport  OutDataTypeStr=double  SampleTime=1/44100  VectorParamsAs1DForOutWhenUnconnected=off
  wires:
  Delay/1 -> Rate Transition/1
  Delay3/1 -> Add/2
  Multiply1/1 -> Delay3/1
  Multiply/1 -> Add/1
  LoD_1/1 -> Multiply/1
  LoD_3/1 -> Multiply1/1
  Add/1 -> Out_LoD_o/1
  In_LoD_o/1 -> Delay/1, Multiply/2
  Rate Transition/1 -> Multiply1/2

== system final_heart_sym2_level4_fixed/1st_Level_Decomp3/HiD_Even ==
  In_HiD_e : Inport  OutDataTypeStr=double  SampleTime=1/44100
  Add : Sum  AccumDataTypeStr=double  OutDataTypeStr=double
  Delay : Delay  DelayLength=1  SampleTime=1/44100
  Delay3 : Delay  DelayLength=1  SampleTime=1/44100
  HiD_0 : Constant  Value=-0.482962913  OutDataTypeStr=double  SampleTime=1/44100
  HiD_2 : Constant  Value=-0.224143868  OutDataTypeStr=double  SampleTime=1/44100
  Multiply : Product  OutDataTypeStr=double
  Multiply1 : Product  OutDataTypeStr=double
  Rate Transition : RateTransition
  Out_HiD_e : Outport  OutDataTypeStr=double  SampleTime=1/44100  VectorParamsAs1DForOutWhenUnconnected=off
  wires:
  Delay/1 -> Rate Transition/1
  Delay3/1 -> Add/2
  Multiply1/1 -> Delay3/1
  Multiply/1 -> Add/1
  HiD_0/1 -> Multiply/1
  HiD_2/1 -> Multiply1/1
  Add/1 -> Out_HiD_e/1
  In_HiD_e/1 -> Multiply/2, Delay/1
  Rate Transition/1 -> Multiply1/2

== system final_heart_sym2_level4_fixed/1st_Level_Decomp3/HiD_Odd ==
  In_HiD_o : Inport  OutDataTypeStr=double  SampleTime=1/44100
  Add : Sum  AccumDataTypeStr=double  OutDataTypeStr=double
  Delay : Delay  DelayLength=1  SampleTime=1/44100
  Delay3 : Delay  DelayLength=1  SampleTime=1/44100
  HiD_1 : Constant  Value=0.836516304  OutDataTypeStr=double  SampleTime=1/44100
  HiD_3 : Constant  Value=-0.129409523  OutDataTypeStr=double  SampleTime=1/44100
  Multiply : Product  OutDataTypeStr=double
  Multiply1 : Product  OutDataTypeStr=double
  Rate Transition : RateTransition
  Out_HiD_o : Outport  OutDataTypeStr=double  SampleTime=1/44100  VectorParamsAs1DForOutWhenUnconnected=off
  wires:
  Delay/1 -> Rate Transition/1
  Delay3/1 -> Add/2
  Multiply1/1 -> Delay3/1
  Multiply/1 -> Add/1
  HiD_1/1 -> Multiply/1
  HiD_3/1 -> Multiply1/1
  Add/1 -> Out_HiD_o/1
  In_HiD_o/1 -> Delay/1, Multiply/2
  Rate Transition/1 -> Multiply1/2

== system final_heart_sym2_level4_fixed/1st_Level_Decomp3/LoD_Even ==
  In_LoD_e : Inport  OutDataTypeStr=double  SampleTime=1/44100
  Add : Sum  AccumDataTypeStr=double  OutDataTypeStr=double
  Delay : Delay  DelayLength=1  SampleTime=1/44100
  Delay3 : Delay  DelayLength=1  SampleTime=1/44100
  LoD_0 : Constant  Value=-0.129409523  OutDataTypeStr=double  SampleTime=1/44100
  LoD_2 : Constant  Value=0.836516304  OutDataTypeStr=double  SampleTime=1/44100
  Multiply : Product  OutDataTypeStr=double
  Multiply1 : Product  OutDataTypeStr=double
  Rate Transition : RateTransition
  Out_LoD_e : Outport  OutDataTypeStr=double  SampleTime=1/44100  VectorParamsAs1DForOutWhenUnconnected=off
  wires:
  Delay/1 -> Rate Transition/1
  Delay3/1 -> Add/2
  Multiply1/1 -> Delay3/1
  Multiply/1 -> Add/1
  LoD_0/1 -> Multiply/1
  LoD_2/1 -> Multiply1/1
  Add/1 -> Out_LoD_e/1
  In_LoD_e/1 -> Delay/1, Multiply/2
  Rate Transition/1 -> Multiply1/2

== system final_heart_sym2_level4_fixed/1st_Level_Decomp3/LoD_Odd ==
  In_LoD_o : Inport  OutDataTypeStr=double  SampleTime=1/44100
  Add : Sum  AccumDataTypeStr=double  OutDataTypeStr=double
  Delay : Delay  DelayLength=1  SampleTime=1/44100
  Delay3 : Delay  DelayLength=1  SampleTime=1/44100
  LoD_1 : Constant  Value=0.224143868  OutDataTypeStr=double  SampleTime=1/44100
  LoD_3 : Constant  Value=0.482962913  OutDataTypeStr=double  SampleTime=1/44100
  Multiply : Product  OutDataTypeStr=double
  Multiply1 : Product  OutDataTypeStr=double
  Rate Transition : RateTransition
  Out_LoD_o : Outport  OutDataTypeStr=double  SampleTime=1/44100  VectorParamsAs1DForOutWhenUnconnected=off
  wires:
  Delay/1 -> Rate Transition/1
  Delay3/1 -> Add/2
  Multiply1/1 -> Delay3/1
  Multiply/1 -> Add/1
  LoD_1/1 -> Multiply/1
  LoD_3/1 -> Multiply1/1
  Add/1 -> Out_LoD_o/1
  In_LoD_o/1 -> Delay/1, Multiply/2
  Rate Transition/1 -> Multiply1/2

== system final_heart_sym2_level4_fixed/1st_Level_Recon/HiR_Even ==
  In_HiR_e : Inport  OutDataTypeStr=double  SampleTime=1/44100
  Add : Sum  AccumDataTypeStr=double  OutDataTypeStr=double
  Constant12 : Constant  Value=-0.129409523  OutDataTypeStr=double  SampleTime=1/44100
  Constant14 : Constant  Value=0.836516304  OutDataTypeStr=double  SampleTime=1/44100
  Delay : Delay  DelayLength=1  SampleTime=1/44100
  Delay3 : Delay  DelayLength=1  SampleTime=1/44100
  Multiply : Product  OutDataTypeStr=double
  Multiply1 : Product  OutDataTypeStr=double
  Rate Transition : RateTransition
  Out_HiR_e : Outport  OutDataTypeStr=double  SampleTime=1/44100  VectorParamsAs1DForOutWhenUnconnected=off
  wires:
  In_HiR_e/1 -> Multiply/2, Delay/1
  Delay3/1 -> Add/2
  Multiply/1 -> Add/1
  Constant12/1 -> Multiply/1
  Constant14/1 -> Multiply1/1
  Delay/1 -> Rate Transition/1
  Multiply1/1 -> Delay3/1
  Add/1 -> Out_HiR_e/1
  Rate Transition/1 -> Multiply1/2

== system final_heart_sym2_level4_fixed/1st_Level_Recon/HiR_Odd ==
  In_HiR_o : Inport  OutDataTypeStr=double  SampleTime=1/44100
  Add : Sum  AccumDataTypeStr=double  OutDataTypeStr=double
  Constant13 : Constant  Value=-0.224143868  OutDataTypeStr=double  SampleTime=1/44100
  Constant15 : Constant  Value=-0.482962913  OutDataTypeStr=double  SampleTime=1/44100
  Delay : Delay  DelayLength=1  SampleTime=1/44100
  Delay3 : Delay  DelayLength=1  SampleTime=1/44100
  Multiply : Product  OutDataTypeStr=double
  Multiply1 : Product  OutDataTypeStr=double
  Rate Transition : RateTransition
  Out_HiR_o : Outport  OutDataTypeStr=double  SampleTime=1/44100  VectorParamsAs1DForOutWhenUnconnected=off
  wires:
  In_HiR_o/1 -> Multiply/2, Delay/1
  Delay3/1 -> Add/2
  Multiply1/1 -> Delay3/1
  Multiply/1 -> Add/1
  Constant13/1 -> Multiply/1
  Constant15/1 -> Multiply1/1
  Add/1 -> Out_HiR_o/1
  Delay/1 -> Rate Transition/1
  Rate Transition/1 -> Multiply1/2

== system final_heart_sym2_level4_fixed/1st_Level_Recon/LoR_Even ==
  In_LoR_e : Inport  OutDataTypeStr=double  SampleTime=1/44100
  Add : Sum  AccumDataTypeStr=double  OutDataTypeStr=double
  Constant10 : Constant  Value=0.224143868  OutDataTypeStr=double  SampleTime=1/44100
  Constant8 : Constant  Value=0.482962913  OutDataTypeStr=double  SampleTime=1/44100
  Delay : Delay  DelayLength=1  SampleTime=1/44100
  Delay3 : Delay  DelayLength=1  SampleTime=1/44100
  Multiply : Product  OutDataTypeStr=double
  Multiply1 : Product  OutDataTypeStr=double
  Rate Transition : RateTransition
  Out_LoR_e : Outport  OutDataTypeStr=double  SampleTime=1/44100  VectorParamsAs1DForOutWhenUnconnected=off
  wires:
  In_LoR_e/1 -> Multiply/2, Delay/1
  Delay3/1 -> Add/2
  Multiply1/1 -> Delay3/1
  Multiply/1 -> Add/1
  Constant8/1 -> Multiply/1
  Constant10/1 -> Multiply1/1
  Add/1 -> Out_LoR_e/1
  Delay/1 -> Rate Transition/1
  Rate Transition/1 -> Multiply1/2

== system final_heart_sym2_level4_fixed/1st_Level_Recon/LoR_Odd ==
  In_LoR_o : Inport  OutDataTypeStr=double  SampleTime=1/44100
  Add : Sum  AccumDataTypeStr=double  OutDataTypeStr=double
  Constant11 : Constant  Value=-0.129409523  OutDataTypeStr=double  SampleTime=1/44100
  Constant9 : Constant  Value=0.836516304  OutDataTypeStr=double  SampleTime=1/44100
  Delay : Delay  DelayLength=1  SampleTime=1/44100
  Delay3 : Delay  DelayLength=1  SampleTime=1/44100
  Multiply : Product  OutDataTypeStr=double
  Multiply1 : Product  OutDataTypeStr=double
  Rate Transition : RateTransition
  Out_HiR_o : Outport  OutDataTypeStr=double  SampleTime=1/44100  VectorParamsAs1DForOutWhenUnconnected=off
  wires:
  In_LoR_o/1 -> Multiply/2, Delay/1
  Delay3/1 -> Add/2
  Multiply1/1 -> Delay3/1
  Multiply/1 -> Add/1
  Constant9/1 -> Multiply/1
  Constant11/1 -> Multiply1/1
  Add/1 -> Out_HiR_o/1
  Delay/1 -> Rate Transition/1
  Rate Transition/1 -> Multiply1/2

== system final_heart_sym2_level4_fixed/1st_Level_Recon1/HiR_Even ==
  In_HiR_e : Inport  OutDataTypeStr=double  SampleTime=1/44100
  Add : Sum  AccumDataTypeStr=double  OutDataTypeStr=double
  Constant12 : Constant  Value=-0.129409523  OutDataTypeStr=double  SampleTime=1/44100
  Constant14 : Constant  Value=0.836516304  OutDataTypeStr=double  SampleTime=1/44100
  Delay : Delay  DelayLength=1  SampleTime=1/44100
  Delay3 : Delay  DelayLength=1  SampleTime=1/44100
  Multiply : Product  OutDataTypeStr=double
  Multiply1 : Product  OutDataTypeStr=double
  Rate Transition : RateTransition
  Out_HiR_e : Outport  OutDataTypeStr=double  SampleTime=1/44100  VectorParamsAs1DForOutWhenUnconnected=off
  wires:
  In_HiR_e/1 -> Multiply/2, Delay/1
  Delay3/1 -> Add/2
  Multiply/1 -> Add/1
  Constant12/1 -> Multiply/1
  Constant14/1 -> Multiply1/1
  Delay/1 -> Rate Transition/1
  Multiply1/1 -> Delay3/1
  Add/1 -> Out_HiR_e/1
  Rate Transition/1 -> Multiply1/2

== system final_heart_sym2_level4_fixed/1st_Level_Recon1/HiR_Odd ==
  In_HiR_o : Inport  OutDataTypeStr=double  SampleTime=1/44100
  Add : Sum  AccumDataTypeStr=double  OutDataTypeStr=double
  Constant13 : Constant  Value=-0.224143868  OutDataTypeStr=double  SampleTime=1/44100
  Constant15 : Constant  Value=-0.482962913  OutDataTypeStr=double  SampleTime=1/44100
  Delay : Delay  DelayLength=1  SampleTime=1/44100
  Delay3 : Delay  DelayLength=1  SampleTime=1/44100
  Multiply : Product  OutDataTypeStr=double
  Multiply1 : Product  OutDataTypeStr=double
  Rate Transition : RateTransition
  Out_HiR_o : Outport  OutDataTypeStr=double  SampleTime=1/44100  VectorParamsAs1DForOutWhenUnconnected=off
  wires:
  In_HiR_o/1 -> Multiply/2, Delay/1
  Delay3/1 -> Add/2
  Multiply1/1 -> Delay3/1
  Multiply/1 -> Add/1
  Constant13/1 -> Multiply/1
  Constant15/1 -> Multiply1/1
  Add/1 -> Out_HiR_o/1
  Delay/1 -> Rate Transition/1
  Rate Transition/1 -> Multiply1/2

== system final_heart_sym2_level4_fixed/1st_Level_Recon1/LoR_Even ==
  In_LoR_e : Inport  OutDataTypeStr=double  SampleTime=1/44100
  Add : Sum  AccumDataTypeStr=double  OutDataTypeStr=double
  Constant10 : Constant  Value=0.224143868  OutDataTypeStr=double  SampleTime=1/44100
  Constant8 : Constant  Value=0.482962913  OutDataTypeStr=double  SampleTime=1/44100
  Delay : Delay  DelayLength=1  SampleTime=1/44100
  Delay3 : Delay  DelayLength=1  SampleTime=1/44100
  Multiply : Product  OutDataTypeStr=double
  Multiply1 : Product  OutDataTypeStr=double
  Rate Transition : RateTransition
  Out_LoR_e : Outport  OutDataTypeStr=double  SampleTime=1/44100  VectorParamsAs1DForOutWhenUnconnected=off
  wires:
  In_LoR_e/1 -> Multiply/2, Delay/1
  Delay3/1 -> Add/2
  Multiply1/1 -> Delay3/1
  Multiply/1 -> Add/1
  Constant8/1 -> Multiply/1
  Constant10/1 -> Multiply1/1
  Add/1 -> Out_LoR_e/1
  Delay/1 -> Rate Transition/1
  Rate Transition/1 -> Multiply1/2

== system final_heart_sym2_level4_fixed/1st_Level_Recon1/LoR_Odd ==
  In_LoR_o : Inport  OutDataTypeStr=double  SampleTime=1/44100
  Add : Sum  AccumDataTypeStr=double  OutDataTypeStr=double
  Constant11 : Constant  Value=-0.129409523  OutDataTypeStr=double  SampleTime=1/44100
  Constant9 : Constant  Value=0.836516304  OutDataTypeStr=double  SampleTime=1/44100
  Delay : Delay  DelayLength=1  SampleTime=1/44100
  Delay3 : Delay  DelayLength=1  SampleTime=1/44100
  Multiply : Product  OutDataTypeStr=double
  Multiply1 : Product  OutDataTypeStr=double
  Rate Transition : RateTransition
  Out_HiR_o : Outport  OutDataTypeStr=double  SampleTime=1/44100  VectorParamsAs1DForOutWhenUnconnected=off
  wires:
  In_LoR_o/1 -> Multiply/2, Delay/1
  Delay3/1 -> Add/2
  Multiply1/1 -> Delay3/1
  Multiply/1 -> Add/1
  Constant9/1 -> Multiply/1
  Constant11/1 -> Multiply1/1
  Add/1 -> Out_HiR_o/1
  Delay/1 -> Rate Transition/1
  Rate Transition/1 -> Multiply1/2

== system final_heart_sym2_level4_fixed/1st_Level_Recon2/HiR_Even ==
  In_HiR_e : Inport  OutDataTypeStr=double  SampleTime=1/44100
  Add : Sum  AccumDataTypeStr=double  OutDataTypeStr=double
  Constant12 : Constant  Value=-0.129409523  OutDataTypeStr=double  SampleTime=1/44100
  Constant14 : Constant  Value=0.836516304  OutDataTypeStr=double  SampleTime=1/44100
  Delay : Delay  DelayLength=1  SampleTime=1/44100
  Delay3 : Delay  DelayLength=1  SampleTime=1/44100
  Multiply : Product  OutDataTypeStr=double
  Multiply1 : Product  OutDataTypeStr=double
  Rate Transition : RateTransition
  Out_HiR_e : Outport  OutDataTypeStr=double  SampleTime=1/44100  VectorParamsAs1DForOutWhenUnconnected=off
  wires:
  In_HiR_e/1 -> Multiply/2, Delay/1
  Delay3/1 -> Add/2
  Multiply/1 -> Add/1
  Constant12/1 -> Multiply/1
  Constant14/1 -> Multiply1/1
  Delay/1 -> Rate Transition/1
  Multiply1/1 -> Delay3/1
  Add/1 -> Out_HiR_e/1
  Rate Transition/1 -> Multiply1/2
